simulink model "VVIBonus"  (R2020a)
settings: Solver=FixedStepAuto  StartTime=0.0  StopTime=10.0  FixedStep=1e-3  RelTol=1e-3  EnableMultiTasking=on
undefined symbols (not defined in the file): D1, D10, D12, D13, D2, D3, D5, D7, D9, PTA1, PTA2, PTB9, PTC17, PTC3, PTC4, PTD0, PTD1, PTD3
libraries: frdmk64flib x12
settings Model: ExtModeTrigDuration=5  Creator=guga  LastModifiedBy=guga
settings OptimizationCC: EnhancedBackFolding=on  PassReuseOutputArgsAs=Individual arguments  ZeroExternalMemoryAtStartup=off  ZeroInternalMemoryAtStartup=off  MaxStackSize=64  OptimizeBlockOrder=speed  DifferentSizesBufferReuse=on  OptimizationCustomize=off  EfficientTunableParamExpr=on
settings DebuggingCC: ParameterTunabilityLossMsg=error
settings HardwareCC: ProdBitPerPointer=32  ProdBitPerSizeT=32  ProdBitPerPtrDiffT=32  ProdLargestAtomicInteger=Long  ProdLargestAtomicFloat=Double  ProdWordSize=32  ProdHWDeviceType=ARM Compatible->ARM Cortex
settings SFSimCC: MATLABDynamicMemAlloc=off
settings RTWCC: SystemTargetFile=ert.tlc  HardwareBoard=NXP FRDM-K64F  TemplateMakefile=ert_default_tmf  Toolchain=GNU Tools for ARM Embedded Processors
settings CodeAppCC: ForceParamTrailComments=on  IgnoreCustomStorageClasses=off  OperatorAnnotations=on  SimulinkDataObjDesc=on  SFDataObjDesc=on  InsertBlockDesc=on

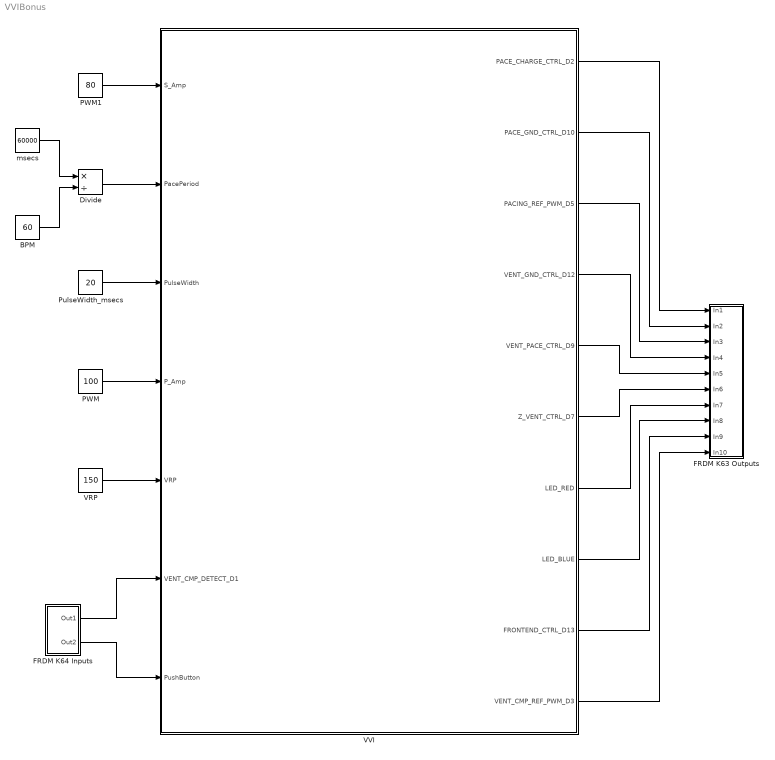
== system VVIBonus ==
  BPM : Constant  Value=60
  Divide : Product  Inputs=*/
  FRDM K63 Outputs : Subsystem
  FRDM K64 Inputs : Subsystem
  PWM : Constant  Value=100
  PWM1 : Constant  Value=80
  PulseWidth_msecs : Constant  Value=20
  VRP : Constant  Value=150
  VVI : Stateflow chart  TreatAsAtomicUnit=on
  msecs : Constant  Value=60000
  wires:
  PWM/1 -> VVI/4(P_Amp)
  PWM1/1 -> VVI/1(S_Amp)
  Divide/1 -> VVI/2(PacePeriod)
  BPM/1 -> Divide/2
  msecs/1 -> Divide/1
  PulseWidth_msecs/1 -> VVI/3(PulseWidth)
  VRP/1 -> VVI/5(VRP)
  FRDM K64 Inputs/1(Out1) -> VVI/6(VENT_CMP_DETECT_D1)
  FRDM K64 Inputs/2(Out2) -> VVI/7(PushButton)
  VVI/1(PACE_CHARGE_CTRL_D2) -> FRDM K63 Outputs/1(In1)
  VVI/2(PACE_GND_CTRL_D10) -> FRDM K63 Outputs/2(In2)
  VVI/3(PACING_REF_PWM_D5) -> FRDM K63 Outputs/3(In3)
  VVI/4(VENT_GND_CTRL_D12) -> FRDM K63 Outputs/4(In4)
  VVI/5(VENT_PACE_CTRL_D9) -> FRDM K63 Outputs/5(In5)
  VVI/6(Z_VENT_CTRL_D7) -> FRDM K63 Outputs/6(In6)
  VVI/7(LED_RED) -> FRDM K63 Outputs/7(In7)
  VVI/8(LED_BLUE) -> FRDM K63 Outputs/8(In8)
  VVI/9(FRONTEND_CTRL_D13) -> FRDM K63 Outputs/9(In9)
  VVI/10(VENT_CMP_REF_PWM_D3) -> FRDM K63 Outputs/10(In10)

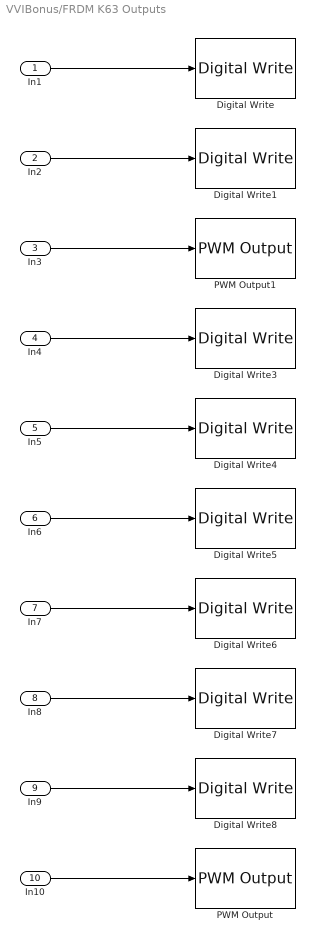
== system VVIBonus/FRDM K63 Outputs ==
  In1 : Inport
  In2 : Inport  Port=2
  In3 : Inport  Port=3
  In4 : Inport  Port=4
  In5 : Inport  Port=5
  In6 : Inport  Port=6
  In7 : Inport  Port=7
  In8 : Inport  Port=8
  In9 : Inport  Port=9
  In10 : Inport  Port=10
  Digital Write : frdmk64flib/Digital Write  Whichpin=PTB9 (D2)
  Digital Write1 : frdmk64flib/Digital Write  Whichpin=PTD0 (D10)
  Digital Write3 : frdmk64flib/Digital Write  Whichpin=PTD3 (D12)
  Digital Write4 : frdmk64flib/Digital Write  Whichpin=PTC4 (D9)
  Digital Write5 : frdmk64flib/Digital Write  Whichpin=PTC3 (D7)
  Digital Write6 : frdmk64flib/Digital Write  Whichpin=RED_LED
  Digital Write7 : frdmk64flib/Digital Write  Whichpin=BLUE_LED
  Digital Write8 : frdmk64flib/Digital Write  Whichpin=PTD1 (D13)
  PWM Output : frdmk64flib/PWM Output  Whichpin=PTA1 (D3)  InitialFrequency=2000  InitialDutyCycle=0
  PWM Output1 : frdmk64flib/PWM Output  Whichpin=PTA2 (D5)  InitialFrequency=2000  InitialDutyCycle=0
  wires:
  In4/1 -> Digital Write3/1
  In2/1 -> Digital Write1/1
  In5/1 -> Digital Write4/1
  In3/1 -> PWM Output1/1
  In8/1 -> Digital Write7/1
  In1/1 -> Digital Write/1
  In6/1 -> Digital Write5/1
  In7/1 -> Digital Write6/1
  In9/1 -> Digital Write8/1
  In10/1 -> PWM Output/1

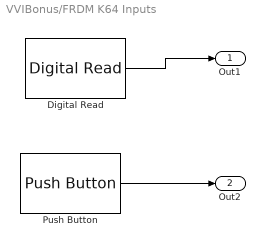
== system VVIBonus/FRDM K64 Inputs ==
  Digital Read : frdmk64flib/Digital Read  Whichpin=PTC17 (D1)  SampleTime=-1
  Push Button : frdmk64flib/Push Button  Whichswitch=SW2  SampleTime1=-1
  Out1 : Outport
  Out2 : Outport  Port=2
  wires:
  Push Button/1 -> Out2/1
  Digital Read/1 -> Out1/1

== stateflow chart VVIBonus/VVI ==
  state Charging_and_Sensing
    entry:
    PACING_REF_PWM_D5 = P_Amp;
    PACE_CHARGE_CTRL_D2 = 1;
    VENT_PACE_CTRL_D9 = 0;
    VENT_GND_CTRL_D12 = 1;
    PACE_GND_CTRL_D10 = 0;
    Z_VENT_CTRL_D7 = 0;
    LED_RED = 0;
    LED_BLUE = 1;
    FRONTEND_CTRL_D13 = 1;
    VENT_CMP_REF_PWM_D3 = S_Amp;
  state Pacing
    entry:
    PACING_REF_PWM_D5 = P_Amp;
    PACE_CHARGE_CTRL_D2 = 0;
    VENT_PACE_CTRL_D9 = 1;
    VENT_GND_CTRL_D12 = 0;
    PACE_GND_CTRL_D10 = 1;
    Z_VENT_CTRL_D7 = 0;
    LED_RED = 1;
    LED_BLUE = 0;
  (junction 22) -> Charging_and_Sensing [order 1] : [VENT_CMP_DETECT_D1 == 1 | PushButton == true]
  (default) -> Charging_and_Sensing
  Charging_and_Sensing -> (junction 22) : after(VRP-PulseWidth,msec)
  (junction 22) -> Pacing [order 2] : after(PacePeriod-VRP,msec)[VENT_CMP_DETECT_D1 == 0 & PushButton == false]
  Pacing -> Charging_and_Sensing : [after(PulseWidth,msec)]
  data: S_Amp input; PacePeriod input; PulseWidth input; P_Amp input; VRP input; VENT_CMP_DETECT_D1 input; PACE_CHARGE_CTRL_D2 output; PACE_GND_CTRL_D10 output; PACING_REF_PWM_D5 output; VENT_GND_CTRL_D12 output; VENT_PACE_CTRL_D9 output; Z_VENT_CTRL_D7 output; LED_RED output; LED_BLUE output; FRONTEND_CTRL_D13 output; VENT_CMP_REF_PWM_D3 output; PushButton input
